simulink model "test"  (R2023b)
settings: Solver=VariableStepAuto  StartTime=0.0  StopTime=100  RelTol=1e-2
values from neighbouring files (symbols this model uses):
  cor_c0 = [40; -26; -15]    [init_para.m]
  cor_d = [2; 0; 0]    [init_para.m]
  k1 = 2.1    [init_para.m]
  k2 = 0.07    [init_para.m]
  k3 = 0.056    [init_para.m]
  k4 = 2    [init_para.m]
  k5 = 0.01    [init_para.m]
  lambda = 0.4    [init_para.m]
  mu = 3.986e14    (= 398600000000000)    [init_para.m]
  r_c0 = (trans_mat*[r_c0;1])    [init_para.m]
  r_t0 = p/(1+e*cos(f)) * A_iL(:,1)    [init_para.m]
  theta = pi/4    (= 0.785398163397)    [init_para.m]
libraries: simulink x1
settings Model: Creator=卢湘骜  LastModifiedBy=卢湘骜

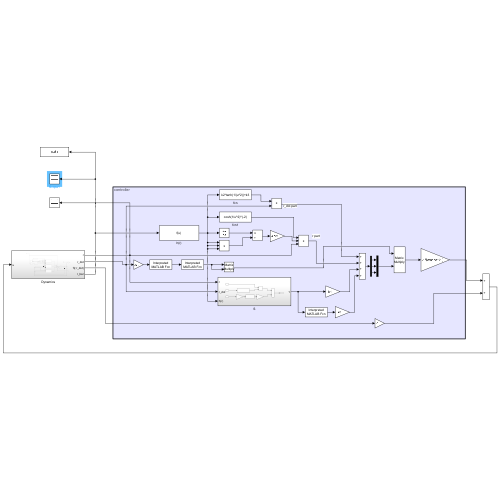
[thumbnail: Simulink's stored preview of the top-level diagram]
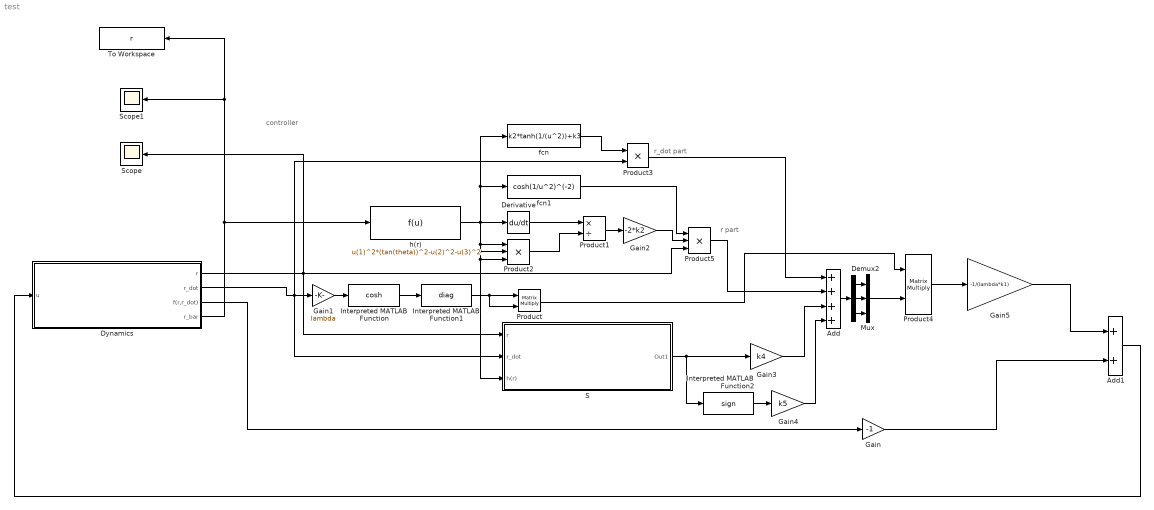
== system test ==
  note: r_dot part
  note: controller
  note: r part
  Add : Sum  Inputs=++++
  Add1 : Sum
  Demux2 : Demux  Outputs=3
  Derivative : Derivative
  Dynamics : Subsystem
  Gain : Gain  Gain=-1
  Gain1 : Gain  Gain=lambda
  Gain2 : Gain  Gain=-2*k2
  Gain3 : Gain  Gain=k4
  Gain4 : Gain  Gain=k5
  Gain5 : Gain  Gain=-1/(lambda*k1)
  Interpreted MATLAB Function : MATLABFcn  MATLABFcn=cosh
  Interpreted MATLAB Function1 : MATLABFcn  MATLABFcn=diag  Output1D=off
  Interpreted MATLAB Function2 : MATLABFcn  MATLABFcn=sign  Output1D=off
  Mux : Mux  Inputs=3
  Product : Product  Multiplication=Matrix(*)
  Product1 : Product  Inputs=*/
  Product2 : Product  Inputs=***
  Product3 : Product  Inputs=**
  Product4 : Product  Multiplication=Matrix(*)
  Product5 : Product  Inputs=***
  S : Subsystem
  Scope : Scope
  Scope1 : Scope
  To Workspace : ToWorkspace  VariableName=r  SampleTime=-1
  fcn : Fcn  Expr=k2*tanh(1/(u^2))+k3
  fcn1 : Fcn  Expr=cosh(1/u^2)^(-2)
  h(r) : Fcn  Expr=u(1)^2*(tan(theta))^2-u(2)^2-u(3)^2
  wires:
  Dynamics/3(f(r,r_dot)) -> Gain/1
  Interpreted MATLAB Function/1 -> Interpreted MATLAB Function1/1
  Interpreted MATLAB Function1/1 -> Product/2, Product/1
  Dynamics/2(r_dot) -> S/2(r_dot), Product3/2, Gain1/1
  Gain1/1 -> Interpreted MATLAB Function/1
  h(r)/1 -> fcn1/1, fcn/1, Derivative/1, Product2/1, S/3(h(r)), Product2/3, Product2/2
  Derivative/1 -> Product1/1
  Product2/1 -> Product1/2
  Product1/1 -> Gain2/1
  Dynamics/1(r) -> Product5/3, Scope/1, S/1(r)
  fcn/1 -> Product3/1
  S/1(Out1) -> Interpreted MATLAB Function2/1, Gain3/1
  Gain3/1 -> Add/3
  Interpreted MATLAB Function2/1 -> Gain4/1
  Gain4/1 -> Add/4
  Product3/1 -> Add/1
  Product/1 -> Product4/1
  Product5/1 -> Add/2
  Product4/1 -> Gain5/1
  Gain5/1 -> Add1/1
  Gain/1 -> Add1/2
  Add1/1 -> Dynamics/1(u)
  Add/1 -> Demux2/1
  Demux2/1 -> Mux/1
  Demux2/2 -> Mux/2
  Demux2/3 -> Mux/3
  Mux/1 -> Product4/2
  Dynamics/4(r_bar) -> To Workspace/1, Scope1/1, h(r)/1
  Gain2/1 -> Product5/2
  fcn1/1 -> Product5/1

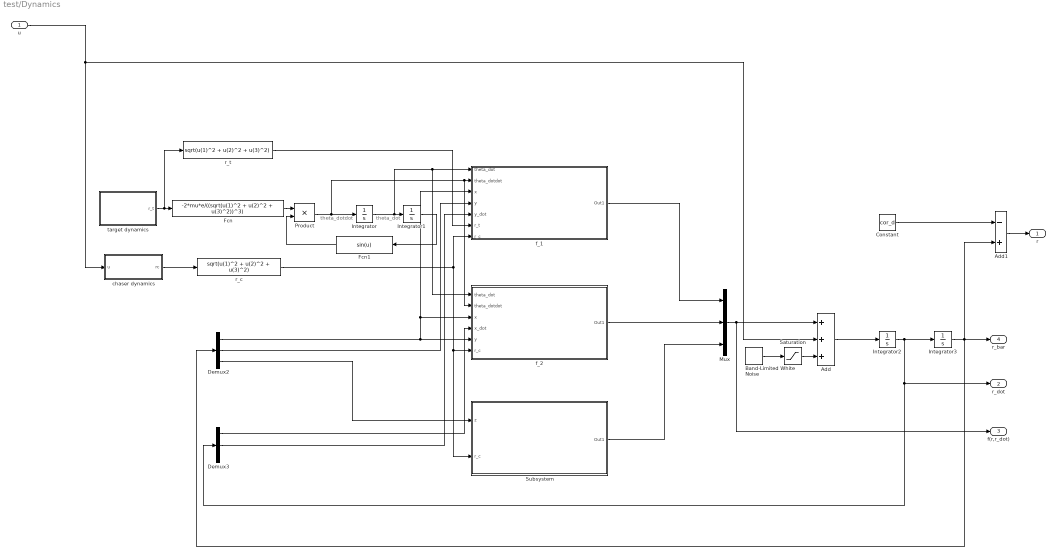
== system test/Dynamics ==
  note: theta_dotdot
  note: theta_dot
  u : Inport
  Add : Sum  Inputs=+++
  Add1 : Sum  Inputs=-+
  Band-Limited White Noise : simulink/Sources/Band-Limited White Noise  Cov=[0.1;0.1;0.1]  Ts=0.1  seed=[23341]
  Constant : Constant  Value=cor_d
  Demux2 : Demux  Outputs=3
  Demux3 : Demux  Outputs=3
  Fcn : Fcn  Expr=-2*mu*e/((sqrt(u(1)^2 + u(2)^2 + u(3)^2))^3)
  Fcn1 : Fcn  Expr=sin(u)
  Integrator : Integrator
  Integrator1 : Integrator
  Integrator2 : Integrator
  Integrator3 : Integrator  InitialCondition=cor_c0
  Mux : Mux  Inputs=3
  Product : Product
  Saturation : Saturate  UpperLimit=0.01  LowerLimit=-0.01
  Subsystem : Subsystem
  chaser dynamics : Subsystem
  f_1 : Subsystem
  f_2 : Subsystem
  r_c : Fcn  Expr=sqrt(u(1)^2 + u(2)^2 + u(3)^2)
  r_t : Fcn  Expr=sqrt(u(1)^2 + u(2)^2 + u(3)^2)
  target dynamics : Subsystem
  r : Outport
  r_dot : Outport  Port=2
  f(r,r_dot) : Outport  Port=3
  r_bar : Outport  Port=4
  wires:
  Integrator/1 -> f_2/1(theta_dot), f_1/1(theta_dot), Integrator1/1
  Integrator1/1 -> Fcn1/1
  target dynamics/1(r_t) -> r_t/1, Fcn/1
  Fcn/1 -> Product/1
  Product/1 -> Integrator/1, f_2/2(theta_dotdot), f_1/2(theta_dotdot)
  Fcn1/1 -> Product/2
  chaser dynamics/1(rc) -> r_c/1
  r_t/1 -> f_1/6(r_t)
  r_c/1 -> f_1/7(r_c), Subsystem/2(r_c), f_2/6(r_c)
  f_1/1(Out1) -> Mux/1
  f_2/1(Out1) -> Mux/2
  Subsystem/1(Out1) -> Mux/3
  Mux/1 -> Add/1, f(r,r_dot)/1
  u/1 -> chaser dynamics/1(u), Add/2
  Add/1 -> Integrator2/1
  Integrator2/1 -> Integrator3/1, Demux3/1, r_dot/1
  Integrator3/1 -> Add1/2, r_bar/1, Demux2/1
  Demux3/1 -> f_2/4(x_dot)
  Demux2/1 -> f_2/3(x), f_1/3(x), f_2/5(y)
  Demux2/2 -> f_1/4(y)
  Demux3/2 -> f_1/5(y_dot)
  Demux2/3 -> Subsystem/1(z)
  Constant/1 -> Add1/1
  Add1/1 -> r/1
  Band-Limited White Noise/1 -> Saturation/1
  Saturation/1 -> Add/3

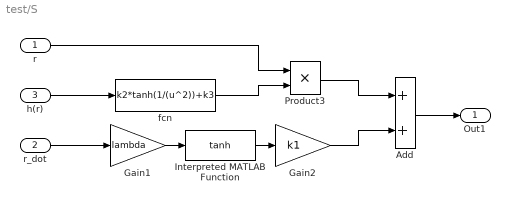
== system test/S ==
  r : Inport
  r_dot : Inport  Port=2
  h(r) : Inport  Port=3
  Add : Sum
  Gain1 : Gain  Gain=lambda
  Gain2 : Gain  Gain=k1
  Interpreted MATLAB Function : MATLABFcn  MATLABFcn=tanh  Output1D=off
  Product3 : Product  Inputs=**
  fcn : Fcn  Expr=k2*tanh(1/(u^2))+k3
  Out1 : Outport
  wires:
  r_dot/1 -> Gain1/1
  r/1 -> Product3/1
  Gain1/1 -> Interpreted MATLAB Function/1
  Interpreted MATLAB Function/1 -> Gain2/1
  h(r)/1 -> fcn/1
  fcn/1 -> Product3/2
  Product3/1 -> Add/1
  Gain2/1 -> Add/2
  Add/1 -> Out1/1

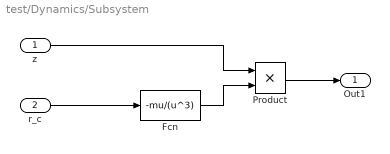
== system test/Dynamics/Subsystem ==
  z : Inport
  r_c : Inport  Port=2
  Fcn : Fcn  Expr=-mu/(u^3)
  Product : Product
  Out1 : Outport
  wires:
  Product/1 -> Out1/1
  r_c/1 -> Fcn/1
  Fcn/1 -> Product/2
  z/1 -> Product/1

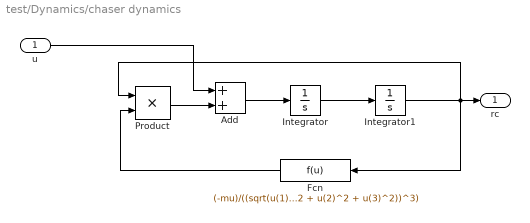
== system test/Dynamics/chaser dynamics ==
  u : Inport
  Add : Sum
  Fcn : Fcn  Expr=(-mu)/((sqrt(u(1)^2 + u(2)^2 + u(3)^2))^3)
  Integrator : Integrator
  Integrator1 : Integrator  InitialCondition=r_c0
  Product : Product
  rc : Outport
  wires:
  Integrator/1 -> Integrator1/1
  Integrator1/1 -> Fcn/1, rc/1, Product/1
  Fcn/1 -> Product/2
  Product/1 -> Add/2
  u/1 -> Add/1
  Add/1 -> Integrator/1

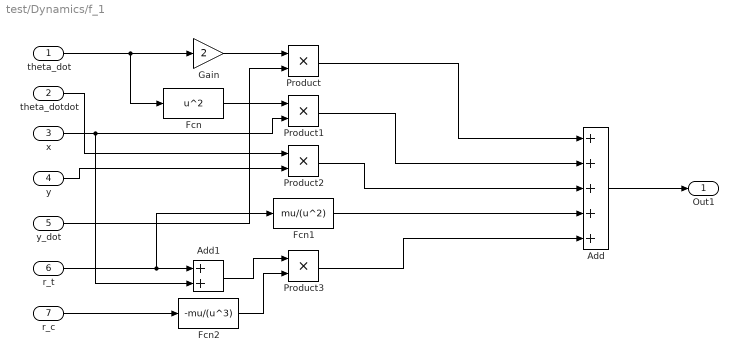
== system test/Dynamics/f_1 ==
  theta_dot : Inport
  theta_dotdot : Inport  Port=2
  x : Inport  Port=3
  y : Inport  Port=4
  y_dot : Inport  Port=5
  r_t : Inport  Port=6
  r_c : Inport  Port=7
  Add : Sum  Inputs=+++++
  Add1 : Sum
  Fcn : Fcn  Expr=u^2
  Fcn1 : Fcn  Expr=mu/(u^2)
  Fcn2 : Fcn  Expr=-mu/(u^3)
  Gain : Gain  Gain=2
  Product{,1..3} (4 alike) : Product
  Out1 : Outport
  wires:
  Gain/1 -> Product/1
  y_dot/1 -> Product/2
  theta_dot/1 -> Fcn/1, Gain/1
  Product/1 -> Add/1
  Fcn/1 -> Product1/1
  x/1 -> Add1/2, Product1/2
  theta_dotdot/1 -> Product2/1
  y/1 -> Product2/2
  r_t/1 -> Fcn1/1, Add1/1
  r_c/1 -> Fcn2/1
  Fcn2/1 -> Product3/2
  Add1/1 -> Product3/1
  Product1/1 -> Add/2
  Product2/1 -> Add/3
  Fcn1/1 -> Add/4
  Product3/1 -> Add/5
  Add/1 -> Out1/1

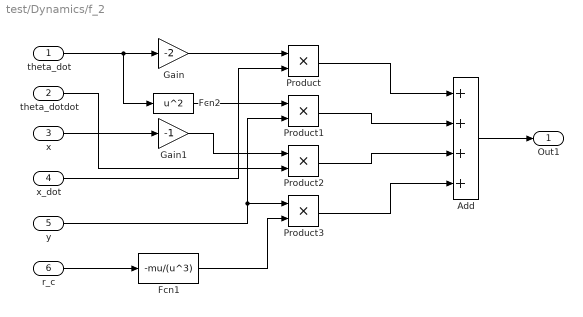
== system test/Dynamics/f_2 ==
  theta_dot : Inport
  theta_dotdot : Inport  Port=2
  x : Inport  Port=3
  x_dot : Inport  Port=4
  y : Inport  Port=5
  r_c : Inport  Port=6
  Add : Sum  Inputs=++++
  Fcn1 : Fcn  Expr=-mu/(u^3)
  Fcn2 : Fcn  Expr=u^2
  Gain : Gain  Gain=-2
  Gain1 : Gain  Gain=-1
  Product{,1..3} (4 alike) : Product
  Out1 : Outport
  wires:
  Add/1 -> Out1/1
  theta_dot/1 -> Fcn2/1, Gain/1
  Gain/1 -> Product/1
  x_dot/1 -> Product/2
  Fcn2/1 -> Product1/1
  y/1 -> Product3/1, Product1/2
  x/1 -> Gain1/1
  Gain1/1 -> Product2/1
  theta_dotdot/1 -> Product2/2
  r_c/1 -> Fcn1/1
  Fcn1/1 -> Product3/2
  Product1/1 -> Add/2
  Product2/1 -> Add/3
  Product3/1 -> Add/4
  Product/1 -> Add/1

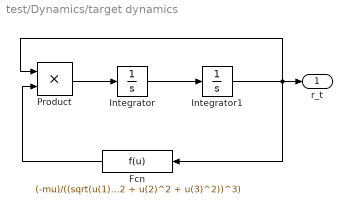
== system test/Dynamics/target dynamics ==
  Fcn : Fcn  Expr=(-mu)/((sqrt(u(1)^2 + u(2)^2 + u(3)^2))^3)
  Integrator : Integrator
  Integrator1 : Integrator  InitialCondition=r_t0
  Product : Product
  r_t : Outport
  wires:
  Integrator/1 -> Integrator1/1
  Product/1 -> Integrator/1
  Fcn/1 -> Product/2
  Integrator1/1 -> r_t/1, Product/1, Fcn/1
